simulink model "FullApp"  (R2015a)
settings: Solver=ode3  StartTime=0.0  StopTime=24.0  RelTol=1e-3
libraries: simulink x1
settings Model: Creator=Morya  LastModifiedBy=Morya
settings OptimizationCC: LifeSpan=1
settings ModelReferenceCC: ModelReferenceNumInstancesAllowed=Single

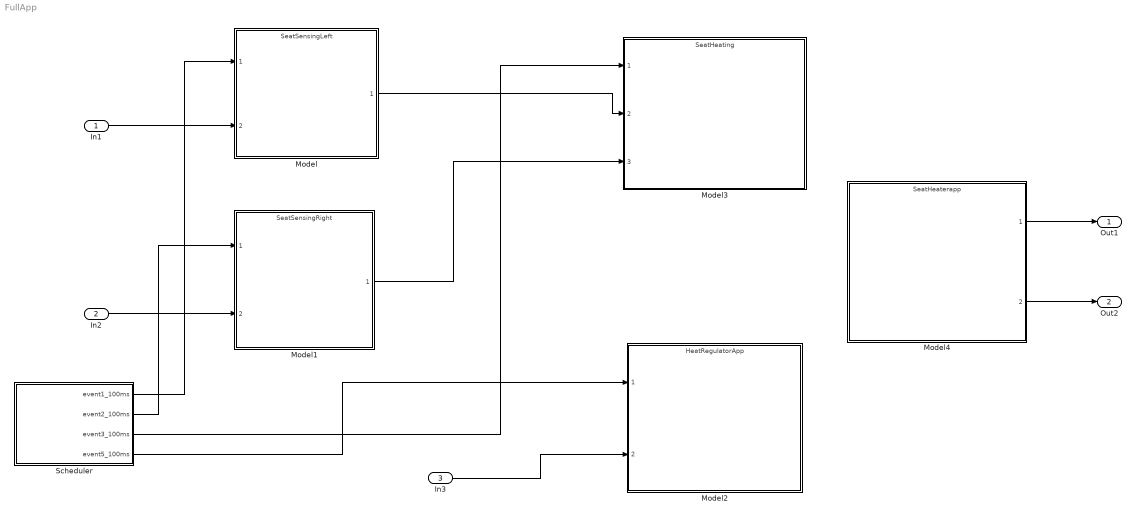
== system FullApp ==
  In1 : Inport
  In2 : Inport  Port=2
  In3 : Inport  Port=3
  Model : ModelReference  ModelNameDialog=SeatSensingLeft.slx  SimulationMode=Normal  ModelReferenceVersion=1.7  CopyOfModelName=SeatSensingLeft.slx  DefaultDataLogging=on
  Model1 : ModelReference  ModelNameDialog=SeatSensingRight.slx  SimulationMode=Normal  ModelReferenceVersion=1.1  CopyOfModelName=SeatSensingRight.slx  DefaultDataLogging=on
  Model2 : ModelReference  ModelNameDialog=HeatRegulatorApp.slx  SimulationMode=Normal  ModelReferenceVersion=1.2  CopyOfModelName=HeatRegulatorApp.slx  DefaultDataLogging=on
  Model3 : ModelReference  ModelNameDialog=SeatHeating.slx  SimulationMode=Normal  ModelReferenceVersion=1.9  CopyOfModelName=SeatHeating.slx  DefaultDataLogging=on
  Model4 : ModelReference  ModelNameDialog=SeatHeaterapp.slx  SimulationMode=Normal  ModelReferenceVersion=1.3  CopyOfModelName=SeatHeaterapp.slx  DefaultDataLogging=on
  "Scheduler " : Subsystem
  Out1 : Outport
  Out2 : Outport  Port=2
  wires:
  "Scheduler "/1(event1_100ms) -> Model/1
  "Scheduler "/2(event2_100ms) -> Model1/1
  "Scheduler "/3("event3_100ms ") -> Model3/1
  "Scheduler "/4("event5_100ms ") -> Model2/1
  Model/1 -> Model3/2
  Model1/1 -> Model3/3
  In2/1 -> Model1/2
  In1/1 -> Model/2
  In3/1 -> Model2/2
  Model4/1 -> Out1/1
  Model4/2 -> Out2/1

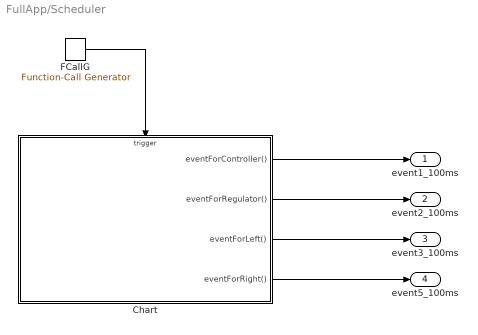
== system FullApp/Scheduler  ==
  Chart : Stateflow chart  TreatAsAtomicUnit=on
  FCallG : simulink/Ports & Subsystems/Function-Call Generator  sample_time=0.1  numberOfIterations=1
  event1_100ms : Outport
  event2_100ms : Outport  Port=2
  "event3_100ms " : Outport  Port=3
  "event5_100ms " : Outport  Port=4
  wires:
  Chart/1(eventForController()) -> event1_100ms/1
  Chart/2(eventForRegulator()) -> event2_100ms/1
  Chart/3(eventForLeft()) -> "event3_100ms "/1
  FCallG/1 -> Chart/Trigger
  Chart/4(eventForRight()) -> "event5_100ms "/1

== stateflow chart FullApp/Scheduler /Chart ==
  state Start
    on every(1,fCallG): send(eventForController);
    on every(1,fCallG): send(eventForRegulator);
    on every(1,fCallG): send(eventForLeft);
    on every(1,fCallG): send(eventForRight);
  (default) -> Start
  events: fCallG input FUNCTION_CALL_EVENT; eventForController output FUNCTION_CALL_EVENT; eventForRegulator output FUNCTION_CALL_EVENT; eventForLeft output FUNCTION_CALL_EVENT; eventForRight output FUNCTION_CALL_EVENT
